simulink model "harness"  (R2019a)
settings: Solver=FixedStepAuto  StartTime=0.0  StopTime=5  FixedStep=T_IR_Plant  RelTol=1e-3
settings Model: Creator=The MathWorks Inc.  LastModifiedBy=seanryu
settings SolverCC: AutoInsertRateTranBlk=on
settings DataIOCC: LimitDataPoints=on  SaveOutput=off  SaveTime=off
settings OptimizationCC: ExpressionDepthLimit=2147483647  LifeSpan=1
settings DebuggingCC: SolverPrmCheckMsg=warning  StateNameClashWarn=warning  SFUnexpectedBacktrackingDiag=warning  SFNoUnconditionalDefaultTransitionDiag=warning  SFExecutionAtInitializationDiag=none  ArithmeticOperatorsInVariantConditions=warning
settings HardwareCC: ProdBitPerPointer=32  ProdBitPerSizeT=32  ProdBitPerPtrDiffT=32  ProdLargestAtomicFloat=None  ProdIntDivRoundTo=Undefined  ProdEndianess=Unspecified  ProdWordSize=32  ProdHWDeviceType=32-bit Generic
settings ModelReferenceCC: ModelReferenceMinAlgLoopOccurrences=on  PropagateSignalLabelsOutOfModel=off
settings SFSimCC: SimUseLocalCustomCode=off
settings RTWCC: RTWUseLocalCustomCode=off
settings CodeAppCC: StateflowObjectComments=on
settings GRTTargetCC: TargetLangStandard=C89/C90 (ANSI)  GeneratePreprocessorConditionals=Disable all  CombineOutputUpdateFcns=off  GRTInterface=on
settings ConfigComp: CovMetricSettings=dw  CovHtmlReporting=on  CovSaveCumulativeToWorkspaceVar=on  CovSaveSingleToWorkspaceVar=on  CovExternalEMLEnable=off

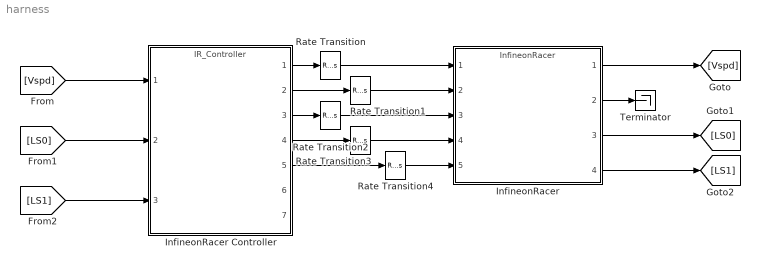
== system harness ==
  InfineonRacer : ModelReference  ModelNameDialog=InfineonRacer.slx  SimulationMode=Normal  ModelReferenceVersion=1.70
  InfineonRacer Controller : ModelReference  ModelNameDialog=IR_Controller  SimulationMode=Normal  ModelReferenceVersion=1.142
  Rate Transition{,1..4} (5 alike) : RateTransition
  Terminator : Terminator
  wires:
  InfineonRacer/1 -> [Vspd]
  InfineonRacer/2 -> Terminator/1
  [Vspd] -> InfineonRacer Controller/1
  InfineonRacer/3 -> [LS0]
  [LS0] -> InfineonRacer Controller/2
  InfineonRacer/4 -> [LS1]
  [LS1] -> InfineonRacer Controller/3
  InfineonRacer Controller/5 -> Rate Transition4/1
  InfineonRacer Controller/2 -> Rate Transition1/1
  InfineonRacer Controller/3 -> Rate Transition2/1
  InfineonRacer Controller/1 -> Rate Transition/1
  InfineonRacer Controller/4 -> Rate Transition3/1
  Rate Transition/1 -> InfineonRacer/1
  Rate Transition1/1 -> InfineonRacer/2
  Rate Transition2/1 -> InfineonRacer/3
  Rate Transition3/1 -> InfineonRacer/4
  Rate Transition4/1 -> InfineonRacer/5
